simulink model "MSFartoystyring"  (R2017b)
settings: Solver=ode45  StartTime=tstart  StopTime=tstop  RelTol=1e-3  EnableMultiTasking=on
values from neighbouring files (symbols this model uses):
  c = 1    [run.m]
  k_d = (2*zeta*sqrt(K*k_p*T) - 1)/K    [task_1_3_.m]
  k_i = 1/T    [task_1_3_.m]
  k_p = w_n^2*T/K    [task_1_3_.m]
  k_ui = 60/T_u    [task_1_7_.m]
  k_up = n_max/e_max    (= 9.89019909463)    [task_1_7_.m]
  p0 = [1000 700]'    [run.m]
  psi0 = 60*deg2rad    (= 1.0471975512)    [run.m]
  r0 = 0    [run.m]
  tsamp = 10    [run.m]
  v0 = [6.63 0]'    [run.m]
undefined symbols (not defined in the file or in its folder): msfartoystyring
settings Model: ExtModeAutoUpdateStatusClock=off  Creator=christh  LastModifiedBy=Ivan
settings DataIOCC: LimitDataPoints=on  SaveFormat=Array  SignalLoggingSaveFormat=ModelDataLogs
settings OptimizationCC: ExpressionDepthLimit=2147483647  InitFltsAndDblsToZero=on  LifeSpan=inf
settings DebuggingCC: UnderspecifiedInitializationDetection=Classic  MergeDetectMultiDrivingBlocksExec=none  SolverPrmCheckMsg=warning  FcnCallInpInsideContextMsg=warning  StateNameClashWarn=warning  SFUnexpectedBacktrackingDiag=warning  SFNoUnconditionalDefaultTransitionDiag=warning  SFExecutionAtInitializationDiag=none
settings HardwareCC: ProdBitPerPointer=32  ProdBitPerSizeT=32  ProdBitPerPtrDiffT=32  ProdLargestAtomicFloat=None  ProdIntDivRoundTo=Undefined  ProdEndianess=Unspecified  ProdWordSize=32  ProdHWDeviceType=32-bit Generic
settings ModelReferenceCC: PropagateSignalLabelsOutOfModel=off
settings CodeAppCC: StateflowObjectComments=on
settings GRTTargetCC: TargetLangStandard=C89/C90 (ANSI)  GeneratePreprocessorConditionals=Disable all  CombineOutputUpdateFcns=off  GRTInterface=on
settings ConfigComp: CovMetricSettings=dw  CovHtmlReporting=on  CovSaveCumulativeToWorkspaceVar=on  CovSaveSingleToWorkspaceVar=on  CovExternalEMLEnable=off

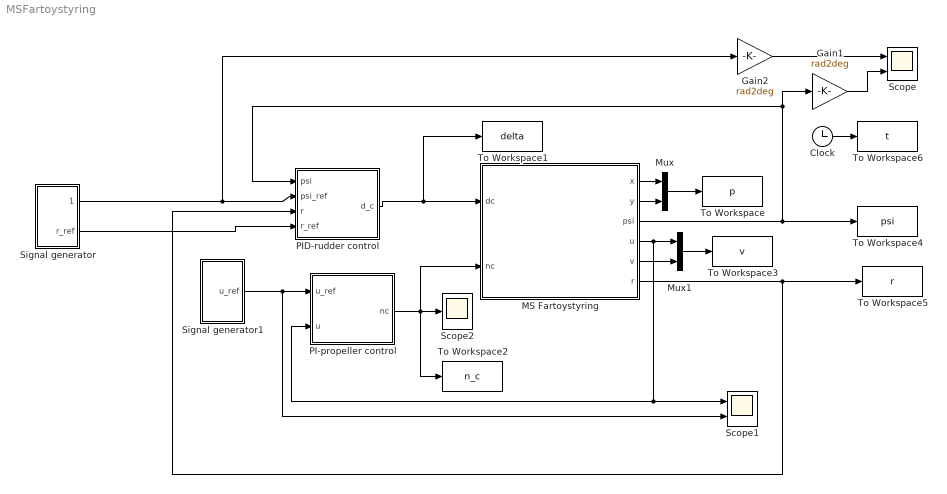
== system MSFartoystyring ==
  Clock : Clock
  Gain1 : Gain  Gain=rad2deg
  Gain2 : Gain  Gain=rad2deg
  MS Fartoystyring : Subsystem  mask(MS Fartoystyring for Assignment 3 G&C){x0=p0(1), y0=p0(2), u0=v0(1), v0=v0(2), psi0=psi0, r0=r0, c=c}
      mask prompts: x0 "x(t0) (m)"; y0 "y(t0) (m)"; u0 "u(t0) (m/s)"; v0 "v(t0) (m/s)"; psi0 "psi(t0) (rad)"; r0 "r(t0) (rad/s)"; c "current (0 or 1)"
      mask help:
      | Block corresponding to Figure 1 in the assignment text. Gives the response of the ship.
      |
      | The design speed of MS Fartoystyring is u=8.23 m/s.
      |
      | Input:
      | dc: commanded rudder (rad), dmax=25*pi/180
      | nc: commanded shaft speed (rad/s), nmax=85*2*pi/60
      |
      | Output:
      | x: north pos (m)
      | y: east pos (m)
      | u: surge (m/s)
      | v: sway (m/s)
      | psi: heading (rad)
      | r: yaw (rad/s)
      mask Help: Comments, bugs and help requests can be directed to the TA. Email on course website.
  Mux : Mux  Inputs=2
  Mux1 : Mux  Inputs=2
  PI-propeller control : Subsystem
  PID-rudder control : Subsystem
  Scope : Scope  NumInputPorts=2
  Scope1 : Scope  NumInputPorts=2
  Scope2 : Scope
  Signal generator : Subsystem
  Signal generator1 : Subsystem
  To Workspace : ToWorkspace  VariableName=p  SampleTime=tsamp
  To Workspace1 : ToWorkspace  VariableName=delta  SaveFormat=Structure With Time  SampleTime=tsamp
  To Workspace2 : ToWorkspace  VariableName=n_c  SampleTime=tsamp
  To Workspace3 : ToWorkspace  VariableName=v  SampleTime=tsamp
  To Workspace4 : ToWorkspace  VariableName=psi  SampleTime=tsamp
  To Workspace5 : ToWorkspace  VariableName=r  SampleTime=tsamp
  To Workspace6 : ToWorkspace  VariableName=t  SampleTime=tsamp
  wires:
  Clock/1 -> To Workspace6/1
  MS Fartoystyring/1(x) -> Mux/1
  MS Fartoystyring/2(y) -> Mux/2
  MS Fartoystyring/4(u) -> PI-propeller control/2(u), Scope1/1, Mux1/1
  MS Fartoystyring/5(v) -> Mux1/2
  Mux/1 -> To Workspace/1
  Mux1/1 -> To Workspace3/1
  MS Fartoystyring/6(r) -> PID-rudder control/3(r), To Workspace5/1
  Signal generator/1(psi_ref) -> Gain2/1, PID-rudder control/2(psi_ref)
  PID-rudder control/1(d_c) -> MS Fartoystyring/1(dc), To Workspace1/1
  Gain1/1 -> Scope/2
  Gain2/1 -> Scope/1
  MS Fartoystyring/3(psi) -> To Workspace4/1, PID-rudder control/1(psi), Gain1/1
  Signal generator1/1(u_ref) -> Scope1/2, PI-propeller control/1(u_ref)
  PI-propeller control/1(nc) -> MS Fartoystyring/2(nc), To Workspace2/1, Scope2/1
  Signal generator/2(r_ref) -> PID-rudder control/4(r_ref)

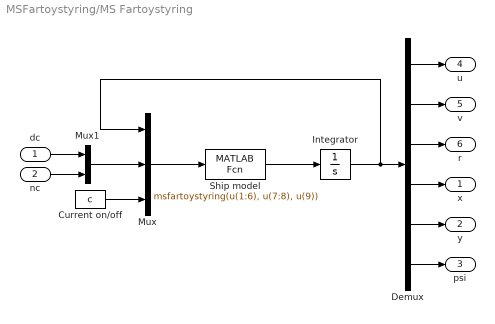
== system MSFartoystyring/MS Fartoystyring ==
  dc : Inport
  nc : Inport  Port=2
  Current on/off : Constant  Value=c
  Demux : Demux  Outputs=6
  Integrator : Integrator  InitialCondition=[u0 v0 r0 x0 y0 psi0]'
  Mux : Mux  Inputs=3
  Mux1 : Mux  Inputs=2
  Ship model : MATLABFcn  MATLABFcn=msfartoystyring(u(1:6), u(7:8), u(9))  OutputDimensions=6
  x : Outport
  y : Outport  Port=2
  psi : Outport  Port=3
  u : Outport  Port=4
  v : Outport  Port=5
  r : Outport  Port=6
  wires:
  Integrator/1 -> Mux/1, Demux/1
  Mux1/1 -> Mux/2
  dc/1 -> Mux1/1
  nc/1 -> Mux1/2
  Demux/1 -> u/1
  Demux/2 -> v/1
  Demux/3 -> r/1
  Demux/4 -> x/1
  Demux/5 -> y/1
  Demux/6 -> psi/1
  Current on/off/1 -> Mux/3
  Ship model/1 -> Integrator/1
  Mux/1 -> Ship model/1

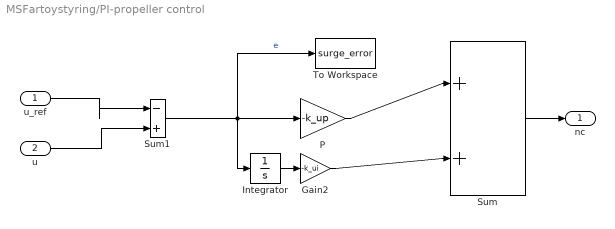
== system MSFartoystyring/PI-propeller control ==
  u_ref : Inport
  u : Inport  Port=2
  Gain2 : Gain  Gain=-k_ui
  Integrator : Integrator
  P : Gain  Gain=-k_up
  Sum : Sum  Inputs=|++
  Sum1 : Sum  Inputs=|-+
  To Workspace : ToWorkspace  VariableName=surge_error  SaveFormat=Structure With Time  SampleTime=tsamp
  nc : Outport
  wires:
  u_ref/1 -> Sum1/1
  Sum1/1 -> To Workspace/1, Integrator/1, P/1  "e"
  P/1 -> Sum/1
  u/1 -> Sum1/2
  Gain2/1 -> Sum/2
  Integrator/1 -> Gain2/1
  Sum/1 -> nc/1

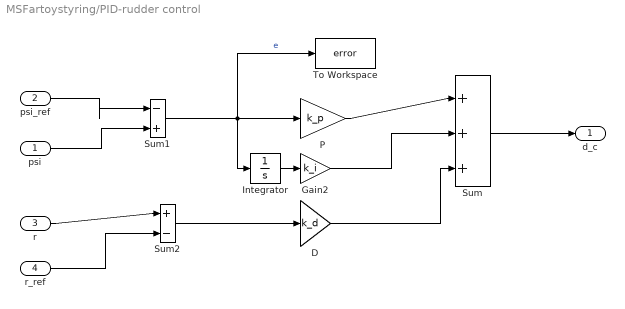
== system MSFartoystyring/PID-rudder control ==
  psi : Inport
  psi_ref : Inport  Port=2
  r : Inport  Port=3
  r_ref : Inport  Port=4
  D : Gain  Gain=k_d
  Gain2 : Gain  Gain=k_i
  Integrator : Integrator
  P : Gain  Gain=k_p
  Sum : Sum  Inputs=|+++
  Sum1 : Sum  Inputs=|-+
  Sum2 : Sum  Inputs=|+-
  To Workspace : ToWorkspace  VariableName=error  SaveFormat=Structure With Time  SampleTime=tsamp
  d_c : Outport
  wires:
  psi_ref/1 -> Sum1/1
  Sum1/1 -> To Workspace/1, Integrator/1, P/1  "e"
  P/1 -> Sum/1
  psi/1 -> Sum1/2
  Gain2/1 -> Sum/2
  D/1 -> Sum/3
  Integrator/1 -> Gain2/1
  Sum/1 -> d_c/1
  r/1 -> Sum2/1
  r_ref/1 -> Sum2/2
  Sum2/1 -> D/1

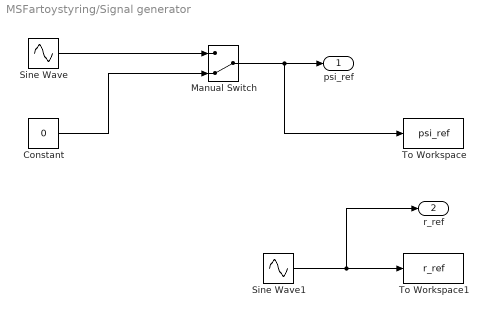
== system MSFartoystyring/Signal generator ==
  Constant : Constant  Value=0
  Manual Switch : ManualSwitch  CurrentSetting=0
  Sine Wave : Sin  Amplitude=0.4  Frequency=0.004  SampleTime=0
  Sine Wave1 : Sin  Amplitude=0.4*0.004  Frequency=0.004  Phase=pi/2  SampleTime=0
  To Workspace : ToWorkspace  VariableName=psi_ref  SaveFormat=Structure With Time  SampleTime=tsamp
  To Workspace1 : ToWorkspace  VariableName=r_ref  SaveFormat=Structure With Time  SampleTime=tsamp
  psi_ref : Outport
  r_ref : Outport  Port=2
  wires:
  Constant/1 -> Manual Switch/2
  Sine Wave/1 -> Manual Switch/1
  Manual Switch/1 -> To Workspace/1, psi_ref/1
  Sine Wave1/1 -> r_ref/1, To Workspace1/1

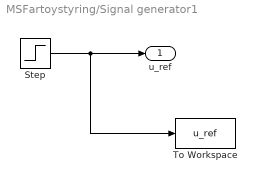
== system MSFartoystyring/Signal generator1 ==
  Step : Step  Time=1250  Before=3  After=5  SampleTime=0
  To Workspace : ToWorkspace  VariableName=u_ref  SaveFormat=Structure With Time  SampleTime=tsamp
  u_ref : Outport
  wires:
  Step/1 -> To Workspace/1, u_ref/1
